simulink model "Simul2"  (R2019b)
settings: Solver=ode4  StartTime=0.0  StopTime=2  FixedStep=0.0005  RelTol=1e-3
values from neighbouring files (symbols this model uses):
  D = 0.003    [parameter.m]
  den_s = [1 2*zeta*omega_s omega_s^2]    [parameter.m]
  Ldelta = 16000    [parameter.m]
  Lp = 3.2    [parameter.m]
  num_s = [omega_s^2]    [parameter.m]
  P = [0.94 0.96 1.00 1.05 1.07 1.09 1.14 1.17 1.21 1.24 1.28]    [HW3_1.m]    (also in parameter.m = 27)
  theta_c = [pi/4 pi/8 0]    [parameter.m]
settings Model: Creator=MoonSunBeen  LastModifiedBy=MoonSunBeen

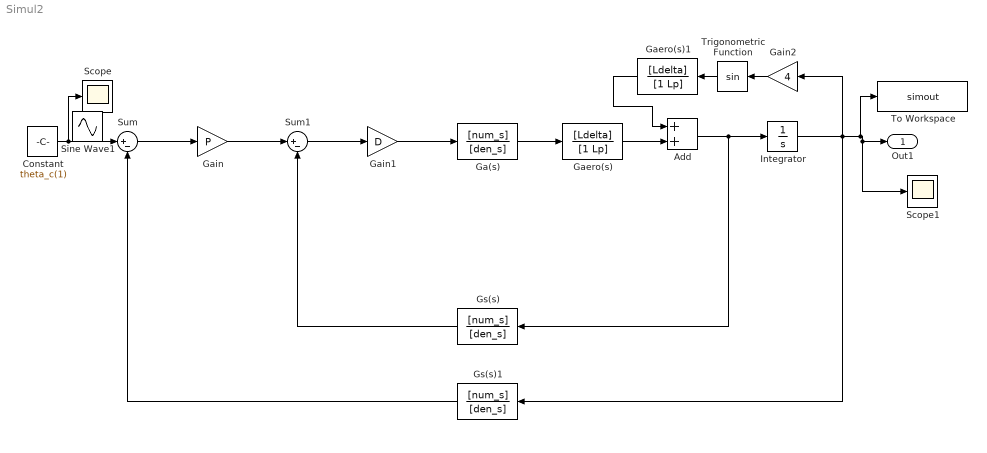
== system Simul2 ==
  Add : Sum
  Constant : Constant  Value=theta_c(1)
  Ga(s) : TransferFcn  Numerator=[num_s]  Denominator=[den_s]
  Gaero(s) : TransferFcn  Numerator=[Ldelta]  Denominator=[1 Lp]
  Gaero(s)1 : TransferFcn  Numerator=[Ldelta]  Denominator=[1 Lp]
  Gain : Gain  Gain=P
  Gain1 : Gain  Gain=D
  Gain2 : Gain  Gain=4
  Gs(s) : TransferFcn  Numerator=[num_s]  Denominator=[den_s]
  Gs(s)1 : TransferFcn  Numerator=[num_s]  Denominator=[den_s]
  Integrator : Integrator
  Scope : Scope
  Scope1 : Scope
  Sum : Sum  Inputs=|+-
  Sum1 : Sum  Inputs=|+-
  To Workspace : ToWorkspace  VariableName=simout  SaveFormat=Timeseries  SampleTime=-1
  Trigonometric Function : Trigonometry
  Out1 : Outport
  Sine Wave1 : Sin  IOType=siggen  SampleTime=0
  wires:
  Sum/1 -> Gain/1
  Gain/1 -> Sum1/1
  Sum1/1 -> Gain1/1
  Gain1/1 -> Ga(s)/1
  Gs(s)/1 -> Sum1/2
  Gs(s)1/1 -> Sum/2
  Constant/1 -> Scope/1, Sum/1
  Integrator/1 -> Gs(s)1/1, Scope1/1, Out1/1, To Workspace/1, Gain2/1
  Gain2/1 -> Trigonometric Function/1
  Add/1 -> Gs(s)/1, Integrator/1
  Gaero(s)/1 -> Add/2
  Ga(s)/1 -> Gaero(s)/1
  Trigonometric Function/1 -> Gaero(s)1/1
  Gaero(s)1/1 -> Add/1
